simulink model "vipsurveillance_fixpt"  (R2020b)
settings: Solver=FixedStepDiscrete  StartTime=0.0  StopTime=inf  RelTol=1e-3
undefined symbols (not defined in the file or in its folder): gray, Rec, SDTV, strel
libraries: visionconversions x3, simulink x2, visiontextngfix x1, visionanalysis x1, visionmorphops x1, dspvision x1
settings Model: FPTRunName=Active  ExtModeAutoUpdateStatusClock=off  Creator=The MathWorks, Inc.  LastModifiedBy=carlo
settings DataIOCC: LimitDataPoints=on  SaveFormat=Array  SaveOutput=off  SaveTime=off  ReturnWorkspaceOutputs=off  SignalLoggingName=sigsOut
settings OptimizationCC: ExpressionDepthLimit=2147483647  InitFltsAndDblsToZero=on  EfficientMapNaN2IntZero=off  LifeSpan=inf
settings DebuggingCC: SaveWithParameterizedLinksMsg=none  UnderspecifiedInitializationDetection=Classic  MergeDetectMultiDrivingBlocksExec=none  CheckExecutionContextPreStartOutputMsg=on  CheckExecutionContextRuntimeOutputMsg=on  SignalResolutionControl=TryResolveAllWithWarning  MultiTaskDSMMsg=warning  ParameterPrecisionLossMsg=none  FcnCallInpInsideContextMsg=warning  StateNameClashWarn=warning  SFUnexpectedBacktrackingDiag=warning  SFNoUnconditionalDefaultTransitionDiag=warning  SFExecutionAtInitializationDiag=none  ArithmeticOperatorsInVariantConditions=warning
settings HardwareCC: ProdBitPerPointer=32  ProdBitPerSizeT=32  ProdBitPerPtrDiffT=32  ProdLargestAtomicFloat=None  ProdIntDivRoundTo=Undefined  ProdEndianess=Unspecified  ProdWordSize=32  ProdHWDeviceType=32-bit Generic  TargetBitPerPointer=64  TargetBitPerSizeT=64  TargetBitPerPtrDiffT=64  TargetLongLongMode=on  TargetIntDivRoundTo=Zero  TargetEndianess=LittleEndian  TargetWordSize=64  TargetHWDeviceType=Generic->MATLAB Host Computer  ProdEqTarget=off
settings ModelReferenceCC: PropagateSignalLabelsOutOfModel=off
settings SFSimCC: SimUseLocalCustomCode=off  CustomCodeUndefinedFunction=UseInterfaceOnly
settings RTWCC: RTWUseLocalCustomCode=off
settings CodeAppCC: StateflowObjectComments=on
settings GRTTargetCC: TargetFcnLib=ansi_tfl_tmw.mat  TargetLangStandard=C89/C90 (ANSI)  CombineOutputUpdateFcns=off  GRTInterface=on
settings ConfigComp: CovMetricSettings=dw  CovSaveCumulativeToWorkspaceVar=on  CovSaveSingleToWorkspaceVar=on  CovExternalEMLEnable=off

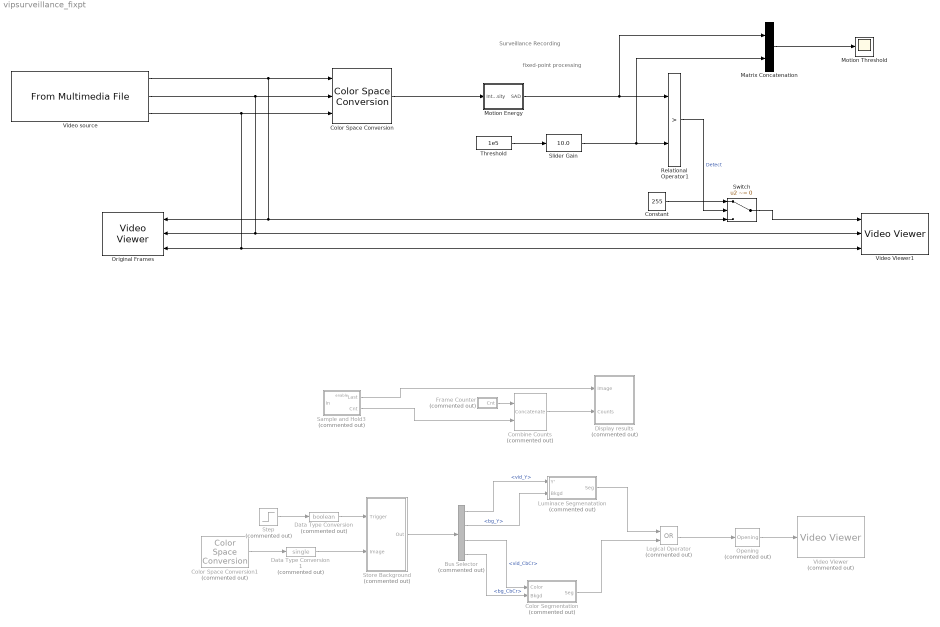
== system vipsurveillance_fixpt ==
  note: Surveillance Recording
  note: fixed-point processing
  Bus Selector : BusSelector  Commented=on  OutputSignals=vid_Y,bg_Y,vid_CbCr,bg_CbCr
  Color Segmentation : Subsystem  Commented=on
      settings: RTWMemSecFuncInitTerm=Default  RTWMemSecFuncExecute=Default  RTWMemSecDataConstants=Default  RTWMemSecDataInternal=Default  RTWMemSecDataParameters=Default
  Color Space Conversion : visionconversions/Color Space  Conversion  conversion=Obsolete  conversionActive=R'G'B' to intensity  wp_str=D65  rec=Rec. 601 (SDTV)  sys=1125/60/2:1  imagePorts=Separate color signals
  Color Space Conversion1 : visionconversions/Color Space  Conversion  Commented=on  conversion=Obsolete  conversionActive=R'G'B' to Y'CbCr  wp_str=D65  rec=Rec. 601 (SDTV)  sys=1125/60/2:1  imagePorts=One multidimensional signal
  Combine Counts : Concatenate  Commented=on  Mode=Multidimensional array  ConcatenateDimension=2
  Constant : Constant  Value=255  OutDataTypeStr=uint8
  Data Type Conversion : DataTypeConversion  Commented=on  OutDataTypeStr=boolean
  Data Type Conversion1 : DataTypeConversion  Commented=on  OutDataTypeStr=single
  Display results : Subsystem  Commented=on
  Frame Counter : Subsystem  Commented=on
  Logical Operator : Logic  Commented=on  Operator=OR  AllPortsSameDT=off  OutDataTypeStr=boolean
  Luminace Segmenatation : Subsystem  Commented=on
      settings: RTWMemSecFuncInitTerm=Default  RTWMemSecFuncExecute=Default  RTWMemSecDataConstants=Default  RTWMemSecDataInternal=Default  RTWMemSecDataParameters=Default
  Matrix Concatenation : Concatenate  Mode=Multidimensional array  ConcatenateDimension=2
  Motion Threshold : Scope
  Motion Energy : Subsystem
  Opening : visionmorphops/Opening  Commented=on  nhoodsrc=Specify via dialog  strel=strel('square',3)
      settings: SourceProductBaseCode=VP
  Original Frames : VideoViewer  imagePorts=separate color signals  colormapValue=gray(256)  FigPos=[-2558 1037 1278 954]  trueSizedOnce=on
  Relational Operator1 : RelationalOperator  Operator=>  OutDataTypeStr=boolean  RndMeth=Nearest  InputSameDT=on
  Sample and Hold3 : Subsystem  Commented=on  TreatAsAtomicUnit=on
  Slider Gain : simulink/Math Operations/Slider Gain  gain=10.0  low=0  high=100
  Step : Step  Commented=on  Time=eps
  Store Background : Subsystem  Commented=on
  Switch : Switch  Criteria=u2 ~= 0  Threshold=1
  Threshold : Constant  Value=1e5  VectorParams1D=off  OutDataTypeStr=Inherit: Inherit via back propagation
  Video Viewer : VideoViewer  Commented=on  FigPos=[2561 1038 1920 938]
  Video Viewer1 : VideoViewer  imagePorts=separate color signals  colormapValue=gray(256)  FigPos=[-1278 1037 1278 929]
  Video source : dspvision/From Multimedia File  inputFilename=D:\3DPrints\Motion_Detection_Camera\VideosRossana\190923_PS\Canon\190923_Canon_PA_visitas.mp4  readRange=[1 Inf]  loop=on  numPlays=inf  outputStreams=Video only  videoDataType=uint8  audioDataType=int16  inheritSampleTime=on  userDefinedSampleTime=1/30  noAudioOutput=off  isIntensityVideo=off  fourcc=RGB  colorVideoFormat=Separate color signals  outputEOF=off  dataOrg=Column-major  audioFrameSize=1024  computeAudioFrameSize=off  outSamplingMode=Frame based
  wires:
  Motion Energy/1(SAD) -> Matrix Concatenation/1, Relational Operator1/1
  Threshold/1 -> Slider Gain/1
  Sample and Hold3/1(Last) -> Display results/1(Image)
  Frame Counter/1(" Cnt") -> Combine Counts/1
  Combine Counts/1 -> Display results/2(Counts)
  Matrix Concatenation/1 -> Motion Threshold/1
  Slider Gain/1 -> Matrix Concatenation/2, Relational Operator1/2
  Sample and Hold3/2(" Cnt") -> Combine Counts/2
  Color Space Conversion1/1 -> Data Type Conversion1/1
  Step/1 -> Data Type Conversion/1
  Data Type Conversion/1 -> Store Background/1(Trigger)
  Logical Operator/1 -> Opening/1
  Bus Selector/2 -> Luminace Segmenatation/2(Bkgd)  "<bg_Y>"
  Luminace Segmenatation/1(Seg) -> Logical Operator/1
  Bus Selector/3 -> Color Segmentation/1(Color)  "<vid_CbCr>"
  Bus Selector/4 -> Color Segmentation/2(Bkgd)  "<bg_CbCr>"
  Color Segmentation/1(Seg) -> Logical Operator/2
  Store Background/1(Out) -> Bus Selector/1
  Bus Selector/1 -> Luminace Segmenatation/1(Y')  "<vid_Y>"
  Data Type Conversion1/1 -> Store Background/2(Image)
  Opening/1 -> Video Viewer/1
  Color Space Conversion/1 -> Motion Energy/1(Intensity)
  Relational Operator1/1 -> Switch/2  "Detect"
  Video source/2 -> Video Viewer1/2, Original Frames/2, Color Space Conversion/2
  Video source/3 -> Original Frames/3, Video Viewer1/3, Color Space Conversion/3
  Constant/1 -> Switch/1
  Video source/1 -> Switch/3, Original Frames/1, Color Space Conversion/1
  Switch/1 -> Video Viewer1/1

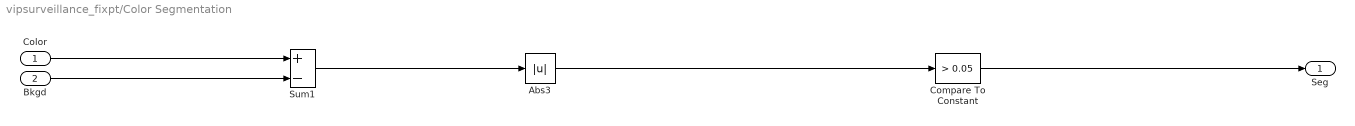
== system vipsurveillance_fixpt/Color Segmentation ==
  Color : Inport
  Bkgd : Inport  Port=2
  Abs3 : Abs  SaturateOnIntegerOverflow=on
  Compare To Constant : simulink/Logic and Bit Operations/Compare To Constant  relop=>  const=0.05  OutDataTypeStr=boolean  ZeroCross=off
  Sum1 : Sum  Inputs=+-  InputSameDT=on  SaturateOnIntegerOverflow=on  OutDataTypeStr=Inherit: Same as first input
  Seg : Outport
  wires:
  Bkgd/1 -> Sum1/2
  Color/1 -> Sum1/1
  Sum1/1 -> Abs3/1
  Compare To Constant/1 -> Seg/1
  Abs3/1 -> Compare To Constant/1

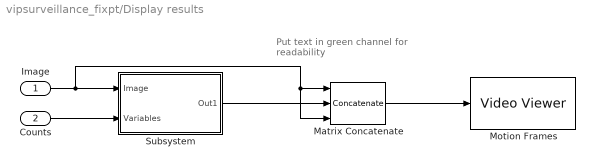
== system vipsurveillance_fixpt/Display results ==
  note: Put text in green
      | channel for readability
  Image : Inport
  Counts : Inport  Port=2
  Matrix Concatenate : Concatenate  NumInputs=3  Mode=Multidimensional array  ConcatenateDimension=3
  Motion Frames : VideoViewer  colormapValue=gray(256)  FigPos=[-1278 1037 1278 954]  trueSizedOnce=on
  Subsystem : Subsystem
  wires:
  Counts/1 -> Subsystem/2(Variables)
  Matrix Concatenate/1 -> Motion Frames/1
  Subsystem/1(Out1) -> Matrix Concatenate/2
  Image/1 -> Matrix Concatenate/1, Matrix Concatenate/3, Subsystem/1(Image)

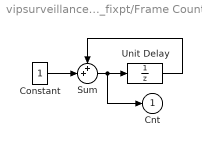
== system vipsurveillance_fixpt/Frame Counter ==
  Constant : Constant  OutDataTypeStr=int32
  Sum : Sum  Inputs=++|  OutDataTypeStr=Inherit: Same as first input
  Unit Delay : UnitDelay  SampleTime=-1  HasFrameUpgradeWarning=on
  " Cnt" : Outport  VectorParamsAs1DForOutWhenUnconnected=off
  wires:
  Constant/1 -> Sum/2
  Sum/1 -> " Cnt"/1, Unit Delay/1
  Unit Delay/1 -> Sum/1

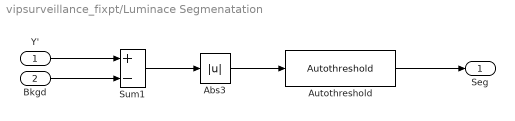
== system vipsurveillance_fixpt/Luminace Segmenatation ==
  Y' : Inport
  Bkgd : Inport  Port=2
  Abs3 : Abs  SaturateOnIntegerOverflow=on
  Autothreshold : visionconversions/Autothreshold  operator=>  threshOut=off  effMetricOut=off  userDefinedRange=off  umin=0  umax=100  outOfRngOpt=Warn and saturate  scaleThreshold=on  scaleFactor=1.3  roundingMode=Floor  overflowMode=off  P1Mode=Specify word length  P1WordLength=32  P1FracLength=30  P2Mode=Specify word length  P2WordLength=32  P2FracLength=22  P3Mode=Specify word length  P3WordLength=32  P3FracLength=14  P4Mode=Binary point scaling  P4WordLength=32  P4FracLength=15  Q1Mode=Specify word length  Q1WordLength=32  Q1FracLength=16  EMMode=Specify word length  EMWordLength=16  EMFracLength=14
      settings: SourceProductBaseCode=VP
  Sum1 : Sum  Inputs=+-  InputSameDT=on  SaturateOnIntegerOverflow=on  OutDataTypeStr=Inherit: Same as first input
  Seg : Outport
  wires:
  Abs3/1 -> Autothreshold/1
  Autothreshold/1 -> Seg/1
  Sum1/1 -> Abs3/1
  Y'/1 -> Sum1/1
  Bkgd/1 -> Sum1/2

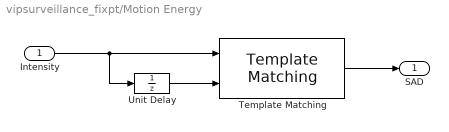
== system vipsurveillance_fixpt/Motion Energy ==
  Intensity : Inport
  Template Matching : visionanalysis/Template Matching  metric=Sum of absolute differences  output=Metric matrix  method=Exhaustive  nMetric=off  nSize=3  roi=off  roiValid=off  roundingMode=Floor  overflowMode=off  prodOutputMode=Binary point scaling  prodOutputWordLength=32  prodOutputFracLength=0  accumMode=Binary point scaling  accumWordLength=23  accumFracLength=0  outputMode=Binary point scaling  outputWordLength=23  outputFracLength=0
      settings: SourceProductBaseCode=VP
  Unit Delay : UnitDelay  SampleTime=-1  HasFrameUpgradeWarning=on
  SAD : Outport  VectorParamsAs1DForOutWhenUnconnected=off
  wires:
  Template Matching/1 -> SAD/1
  Intensity/1 -> Template Matching/1, Unit Delay/1
  Unit Delay/1 -> Template Matching/2

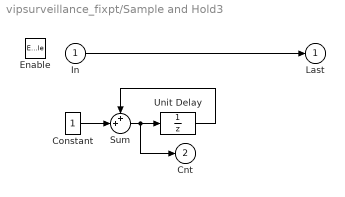
== system vipsurveillance_fixpt/Sample and Hold3 ==
  In : Inport
  Enable : EnablePort  PropagateVarSize=During execution
  Constant : Constant  OutDataTypeStr=int32
  Sum : Sum  Inputs=++|  OutDataTypeStr=Inherit: Same as first input
  Unit Delay : UnitDelay  SampleTime=-1  HasFrameUpgradeWarning=on
  Last : Outport  VectorParamsAs1DForOutWhenUnconnected=off
  " Cnt" : Outport  Port=2  VectorParamsAs1DForOutWhenUnconnected=off
  wires:
  Unit Delay/1 -> Sum/1
  Sum/1 -> " Cnt"/1, Unit Delay/1
  Constant/1 -> Sum/2
  In/1 -> Last/1

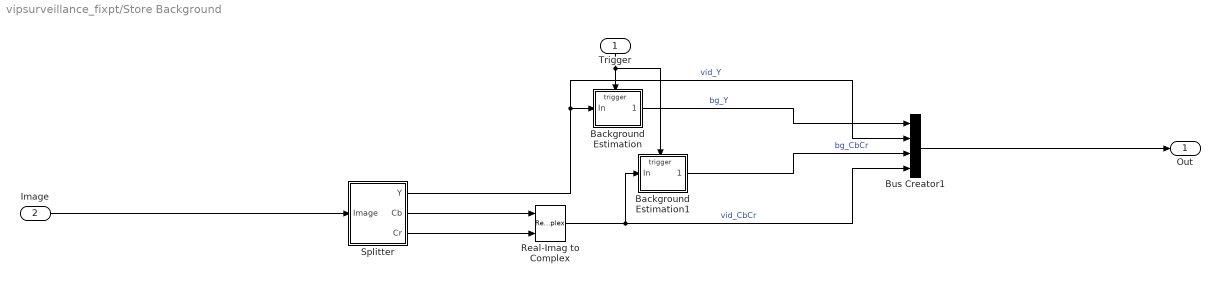
== system vipsurveillance_fixpt/Store Background ==
  Trigger : Inport
  Image : Inport  Port=2
  Background Estimation : Subsystem  TreatAsAtomicUnit=on  mask{initCond=0}
      mask prompts: initCond "Initial Condition"
  Background Estimation1 : Subsystem  TreatAsAtomicUnit=on  mask{initCond=0}
      mask prompts: initCond "Initial Condition"
  Bus Creator1 : BusCreator  Inputs=4
  Real-Imag to Complex : RealImagToComplex
  Splitter : Subsystem
  Out : Outport
  wires:
  Image/1 -> Splitter/1(Image)
  Splitter/3(Cr) -> Real-Imag to Complex/2
  Splitter/2(Cb) -> Real-Imag to Complex/1
  Bus Creator1/1 -> Out/1
  Trigger/1 -> Background Estimation/Trigger, Background Estimation1/Trigger
  Background Estimation1/1(" ") -> Bus Creator1/3  "bg_CbCr"
  Background Estimation/1(" ") -> Bus Creator1/1  "bg_Y"
  Real-Imag to Complex/1 -> Bus Creator1/4, Background Estimation1/1(In)  "vid_CbCr"
  Splitter/1(Y) -> Bus Creator1/2, Background Estimation/1(In)  "vid_Y"

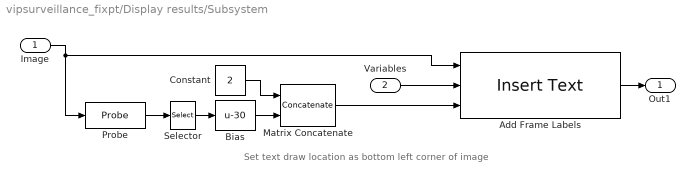
== system vipsurveillance_fixpt/Display results/Subsystem ==
  note: Set text draw location as bottom left corner of image
  Image : Inport
  Variables : Inport  Port=2
  Add Frame Labels : visiontextngfix/Insert Text  inputType=Obsolete  theText=['Source frame: %d' sprintf('\n') 'Captured frame: %d']  getTextLocFrom=Input port  textLoc=[90 2]  getTextColorFrom=Specify via dialog  textColor=255  getTextIntensityFrom=Specify via dialog  textIntensity=1  getTextOpacityFrom=Specify via dialog  textOpacity=1.0  dummyVar2=0  dummyVar3=0  dummyVar4=0  imagePorts=One multidimensional signal  isInputTransposed=off  fontFace=LucidaTypewriterRegular  dummyVar1=0  blockFontSize=12  antiAliased=on
      settings: SourceProductBaseCode=VP
  Bias : Bias  Bias=-30
  Constant : Constant  Value=2  OutDataTypeStr=int32
  Matrix Concatenate : Concatenate  Mode=Multidimensional array  ConcatenateDimension=2
  Probe : Probe  ProbeWidth=off  ProbeSampleTime=off  ProbeComplexSignal=off  ProbeSignalDimensions=on  ProbeDimensionsDataType=int32
  Selector : Selector  InputPortWidth=2  IndexOptions=Index vector (dialog)  Indices=1  OutputSizes=1
  Out1 : Outport  VectorParamsAs1DForOutWhenUnconnected=off
  wires:
  Constant/1 -> Matrix Concatenate/1
  Bias/1 -> Matrix Concatenate/2
  Image/1 -> Add Frame Labels/1, Probe/1
  Variables/1 -> Add Frame Labels/2
  Add Frame Labels/1 -> Out1/1
  Probe/1 -> Selector/1
  Selector/1 -> Bias/1
  Matrix Concatenate/1 -> Add Frame Labels/3

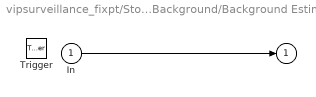
== system vipsurveillance_fixpt/Store Background/Background Estimation ==
  In : Inport
  Trigger : TriggerPort  VariantControl=(inherit)  ZeroCross=off
  " " : Outport  InitialOutput=initCond
  wires:
  In/1 -> " "/1

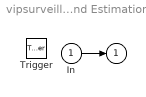
== system vipsurveillance_fixpt/Store Background/Background Estimation1 ==
  In : Inport
  Trigger : TriggerPort  VariantControl=(inherit)  ZeroCross=off
  " " : Outport  InitialOutput=initCond
  wires:
  In/1 -> " "/1

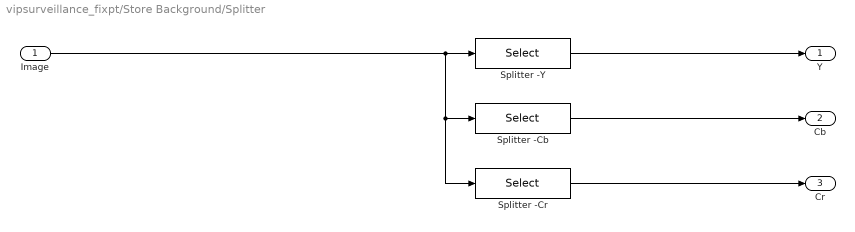
== system vipsurveillance_fixpt/Store Background/Splitter ==
  Image : Inport
  Splitter -Cb : Selector  NumberOfDimensions=3  IndexOptions=Select all,Select all,Index vector (dialog)  Indices=[],[],[2]  OutputSizes=1
  Splitter -Cr : Selector  NumberOfDimensions=3  IndexOptions=Select all,Select all,Index vector (dialog)  Indices=[],[],[3]  OutputSizes=1
  Splitter -Y : Selector  NumberOfDimensions=3  IndexOptions=Select all,Select all,Index vector (dialog)  Indices=[],[],[1]  OutputSizes=1
  Y : Outport
  Cb : Outport  Port=2
  Cr : Outport  Port=3
  wires:
  Image/1 -> Splitter -Cr/1, Splitter -Cb/1, Splitter -Y/1
  Splitter -Y/1 -> Y/1
  Splitter -Cb/1 -> Cb/1
  Splitter -Cr/1 -> Cr/1
